simulink model "mod7"  (R2022a)
settings: Solver=FixedStepDiscrete  StartTime=0.0  StopTime=inf  FixedStep=0.01  RelTol=1e-3
values from neighbouring files (symbols this model uses):
  DD = 3.0    [data1.sldd]
  NN = 2.0    [data1.sldd]
  PP = 0.0    [data1.sldd]
  RR = 1.0    [data1.sldd]
settings Model: DataDictionary=data1.sldd  Creator=Administrator  LastModifiedBy=Administrator
settings OptimizationCC: DefaultParameterBehavior=Inlined  EnhancedBackFolding=on  PassReuseOutputArgsAs=Individual arguments  ZeroExternalMemoryAtStartup=off  ZeroInternalMemoryAtStartup=off  OptimizeBlockOrder=speed  DifferentSizesBufferReuse=on  OptimizationCustomize=off  EfficientTunableParamExpr=on
settings DebuggingCC: ParameterTunabilityLossMsg=error
settings SFSimCC: MATLABDynamicMemAlloc=off
settings RTWCC: SystemTargetFile=ert.tlc  TemplateMakefile=ert_default_tmf  GenerateReport=on  LaunchReport=on
settings CodeAppCC: ForceParamTrailComments=on  IgnoreCustomStorageClasses=off  OperatorAnnotations=on  SimulinkDataObjDesc=on  SFDataObjDesc=on  InsertBlockDesc=on
settings ERTTargetCC: TargetLangStandard=C99 (ISO)  GenerateSampleERTMain=on  SupportContinuousTime=on  InlinedParameterPlacement=NonHierarchical  ERTCustomFileTemplate=example_file_process.tlc

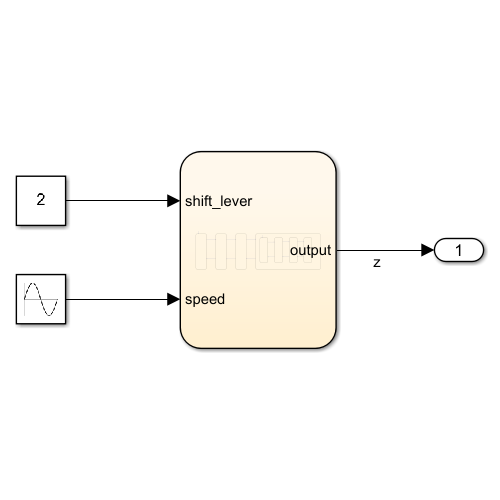
[thumbnail: Simulink's stored preview of the top-level diagram]
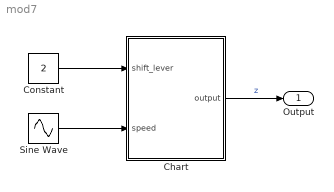
== system mod7 ==
  Chart : Stateflow chart  TreatAsAtomicUnit=on
  Constant : Constant  Value=2
  Sine Wave : Sin  Amplitude=100  SampleTime=0
  Output : Outport
  wires:
  Chart/1(output) -> Output/1  "z"
  Sine Wave/1 -> Chart/2(speed)
  Constant/1 -> Chart/1(shift_lever)

== stateflow chart mod7/Chart ==
  state P
  state R
  state N
  state D
    state D1
      en:
      output = 10;
      du:
      output = 20;
      ex:
      output = 30;
    state D2
      en:
      output = 20;
    state D3
      en:
      output = 30;
    state D4
      en:
      output = 40;
    (default) -> D1
    D2 -> D3 [order 1] : [speed>50]
    D3 -> D4 [order 1] : [speed>70]
    D1 -> D2 : [speed>30]
    D4 -> D3 : [speed<65]
    D3 -> D2 [order 2] : [speed<45]
    D2 -> D1 [order 2] : [speed<25]
  (default) -> P
  N -> D [order 1] : [shift_lever==DD]
  R -> N [order 1] : [shift_lever==NN]
  P -> R : [shift_lever==RR]
  D -> N : [shift_lever==NN]
  R -> P [order 2] : [shift_lever==PP]
  N -> R [order 2] : [shift_lever==RR]
  data: shift_lever input; output output; speed input; RR parameter; NN parameter; DD parameter; PP parameter
